simulink model "MotorControl_Bldc"  (R2022a)
settings: Solver=ode4  StartTime=0.0  StopTime=1  FixedStep=Ts/cnt_pTs  RelTol=1e-3
values from neighbouring files (symbols this model uses):
  cnt_pTs = 1000    [motorpara.m]
  Fc = 1/Ts    (= 10000)    [motorpara.m]
  Ki_id = Rs*Fc    (= 4500)    [motorpara.m]
  Ki_iq = Rs*Fc    (= 4500)    [motorpara.m]
  Ki_v = 0.93    [motorpara.m]
  Kp_id = Ls*Fc    (= 4.2)    [motorpara.m]
  Kp_iq = Ls*Fc    (= 4.2)    [motorpara.m]
  Kp_v = 0.05    [motorpara.m]
  Ls = 0.00042    [motorpara.m]
  P = 2    [motorpara.m]
  Rs = 0.45    [motorpara.m]
  SMO_Kslide = 10    [motorpara.m]
  Ts = 1/10000    (= 0.0001)    [motorpara.m]
  V = 12    [motorpara.m]
undefined symbols (not defined in the file or in its folder): DiscIntNeverNeededParam, sigbuilder_block
libraries: nesl_utility x83, fl_lib x67, ee_lib x49, simulink x13, slpidlib x3, mcbplantlib x2, autolibpmsmexterior x1
(part 2 of 4)

== system MotorControl_Bldc/2Phase_D1D1 ==
  alpha : Inport
  m : Inport  Port=2
  N : Inport  Port=3
  Cos : Trigonometry  Operator=cos
  Index Vector : MultiPortSwitch  Inputs=6  DiagnosticForDefault=None  SaturateOnIntegerOverflow=off  InputSameDT=off
  Index Vector1 : MultiPortSwitch  Inputs=6  DiagnosticForDefault=None  SaturateOnIntegerOverflow=off  InputSameDT=off
  Sin : Trigonometry
  c_s : Sum  Inputs=+-
  mcos : Product
  mcos_ : Gain  Gain=-1
  msin : Product
  msin_ : Gain  Gain=-1
  s_c : Gain  Gain=-1
  D1 : Outport
  D2 : Outport  Port=2
  wires:
  Index Vector1/1 -> D2/1
  N/1 -> Index Vector1/1, Index Vector/1
  Index Vector/1 -> D1/1
  alpha/1 -> Sin/1, Cos/1
  Sin/1 -> msin/2
  Cos/1 -> mcos/1
  m/1 -> mcos/2, msin/1
  mcos/1 -> Index Vector/7, Index Vector/3, mcos_/1, c_s/1
  msin/1 -> msin_/1, c_s/2, Index Vector/4, Index Vector1/2
  c_s/1 -> Index Vector1/6, Index Vector/2, s_c/1
  s_c/1 -> Index Vector/5, Index Vector1/3
  mcos_/1 -> Index Vector/6, Index Vector1/4
  msin_/1 -> Index Vector1/7, Index Vector1/5

== system MotorControl_Bldc/2Phase_D1D1_org ==
  alpha : Inport
  m : Inport  Port=2
  N : Inport  Port=3
  Cos : Trigonometry  Operator=cos
  Index Vector : MultiPortSwitch  Inputs=6  DiagnosticForDefault=None  SaturateOnIntegerOverflow=off  InputSameDT=off
  Index Vector1 : MultiPortSwitch  Inputs=6  DiagnosticForDefault=None  SaturateOnIntegerOverflow=off  InputSameDT=off
  Sin : Trigonometry
  c_s : Sum  Inputs=+-
  mcos : Product
  mcos_ : Gain  Gain=-1
  msin : Product
  msin_ : Gain  Gain=-1
  s_c : Gain  Gain=-1
  D1 : Outport
  D2 : Outport  Port=2
  wires:
  Index Vector1/1 -> D2/1
  N/1 -> Index Vector1/1, Index Vector/1
  Index Vector/1 -> D1/1
  alpha/1 -> Sin/1, Cos/1
  Sin/1 -> msin/2
  Cos/1 -> mcos/1
  m/1 -> mcos/2, msin/1
  mcos/1 -> Index Vector/7, Index Vector/3, mcos_/1, c_s/1
  msin/1 -> msin_/1, c_s/2, Index Vector1/7, Index Vector/4, Index Vector1/2
  c_s/1 -> Index Vector1/6, Index Vector/5, Index Vector/2, s_c/1
  s_c/1 -> Index Vector1/3
  mcos_/1 -> Index Vector/6, Index Vector1/4
  msin_/1 -> Index Vector1/5

== system MotorControl_Bldc/2Phase_D1D2 ==
  alpha : Inport
  m : Inport  Port=2
  N : Inport  Port=3
  Cos : Trigonometry  Operator=cos
  Index Vector : MultiPortSwitch  Inputs=6  DiagnosticForDefault=None  SaturateOnIntegerOverflow=off  InputSameDT=off
  Index Vector1 : MultiPortSwitch  Inputs=6  DiagnosticForDefault=None  SaturateOnIntegerOverflow=off  InputSameDT=off
  Sin : Trigonometry
  c_s : Sum  Inputs=+-
  mcos : Product
  mcos_ : Gain  Gain=-1
  msin : Product
  msin_ : Gain  Gain=-1
  s_c : Gain  Gain=-1
  D1 : Outport
  D2 : Outport  Port=2
  wires:
  Index Vector1/1 -> D2/1
  N/1 -> Index Vector1/1, Index Vector/1
  Index Vector/1 -> D1/1
  alpha/1 -> Sin/1, Cos/1
  Sin/1 -> msin/2
  Cos/1 -> mcos/1
  m/1 -> mcos/2, msin/1
  mcos/1 -> Index Vector1/7, Index Vector/3, mcos_/1, c_s/1
  msin/1 -> msin_/1, c_s/2, Index Vector/4, Index Vector1/2
  c_s/1 -> Index Vector1/6, Index Vector/2, s_c/1
  s_c/1 -> Index Vector/5, Index Vector1/3
  mcos_/1 -> Index Vector/6, Index Vector1/4
  msin_/1 -> Index Vector/7, Index Vector1/5

== system MotorControl_Bldc/2Phase_T ==
  note: D1+D2
  note: D1
  note: 1-D1
  note: 1-D1-D2
  N : Inport
  D1 : Inport  Port=2
  D2 : Inport  Port=3
  1_t1 : Sum  Inputs=-+
  1_t2_T2 : Sum  Inputs=-+
  Constant : Constant
  Constant1 : Constant  Value=0
  Index Vector : MultiPortSwitch  Inputs=6  DiagnosticForDefault=None  SaturateOnIntegerOverflow=off  InputSameDT=off
  Index Vector1 : MultiPortSwitch  Inputs=6  DiagnosticForDefault=None  SaturateOnIntegerOverflow=off  InputSameDT=off
  Index Vector2 : MultiPortSwitch  Inputs=6  DiagnosticForDefault=None  SaturateOnIntegerOverflow=off  InputSameDT=off
  T1AT2 : Sum
  Da : Outport
  Db : Outport  Port=2
  Dc : Outport  Port=3
  wires:
  D1/1 -> Index Vector/3, Index Vector2/7, Index Vector1/5, 1_t1/1, T1AT2/1
  D2/1 -> 1_t2_T2/1, T1AT2/2
  N/1 -> Index Vector2/1, Index Vector1/1, Index Vector/1
  Index Vector/1 -> Da/1
  Index Vector1/1 -> Db/1
  Index Vector2/1 -> Dc/1
  Constant/1 -> Index Vector2/6, Index Vector1/4, Index Vector/2, 1_t1/2
  1_t1/1 -> Index Vector1/2, Index Vector/6, Index Vector2/4, 1_t2_T2/2
  T1AT2/1 -> Index Vector/7, Index Vector1/3, Index Vector2/5
  Constant1/1 -> Index Vector1/7, Index Vector/5, Index Vector2/3
  1_t2_T2/1 -> Index Vector2/2, Index Vector1/6, Index Vector/4

== system MotorControl_Bldc/Duty_conver ==
  In1 : Inport
  Constant : Constant  Value=0.5
  Gain : Gain  Gain=1/(5e-5)
  Gain1 : Gain  Gain=-1
  Sum : Sum  Inputs=|+-
  Sum1 : Sum  Inputs=|++
  Out1 : Outport
  wires:
  In1/1 -> Gain/1
  Gain/1 -> Sum/1
  Sum/1 -> Gain1/1
  Gain1/1 -> Sum1/1
  Sum1/1 -> Out1/1
  Constant/1 -> Sum1/2, Sum/2

== system MotorControl_Bldc/Duty_conver1 ==
  In1 : Inport
  Constant : Constant  Value=0.5
  Gain : Gain  Gain=2
  Gain1 : Gain  Gain=-1
  Sum : Sum  Inputs=|+-
  Sum1 : Sum  Inputs=|++
  Out1 : Outport
  wires:
  In1/1 -> Gain/1
  Gain/1 -> Sum/1
  Sum/1 -> Gain1/1
  Gain1/1 -> Sum1/1
  Sum1/1 -> Out1/1
  Constant/1 -> Sum1/2, Sum/2

== system MotorControl_Bldc/Inverse_Park ==
  Vd : Inport
  Vq : Inport  Port=2
  sin_theta : Inport  Port=3
  cos_theta : Inport  Port=4
  Add : Sum  Inputs=+-
  Add1 : Sum
  Product{,1..3} (4 alike) : Product
  Vα : Outport
  Vβ : Outport  Port=2
  wires:
  Vd/1 -> Product3/1, Product/1
  cos_theta/1 -> Product2/2, Product/2
  Vq/1 -> Product2/1, Product1/1
  sin_theta/1 -> Product3/2, Product1/2
  Product/1 -> Add/1
  Product1/1 -> Add/2
  Add/1 -> Vα/1
  Product2/1 -> Add1/1
  Product3/1 -> Add1/2
  Add1/1 -> Vβ/1

== system MotorControl_Bldc/Inverse_Park1 ==
  Vd : Inport
  Vq : Inport  Port=2
  sin_theta : Inport  Port=3
  cos_theta : Inport  Port=4
  Add : Sum  Inputs=+-
  Add1 : Sum
  Product{,1..3} (4 alike) : Product
  Vα : Outport
  Vβ : Outport  Port=2
  wires:
  Vd/1 -> Product3/1, Product/1
  cos_theta/1 -> Product2/2, Product/2
  Vq/1 -> Product2/1, Product1/1
  sin_theta/1 -> Product3/2, Product1/2
  Product/1 -> Add/1
  Product1/1 -> Add/2
  Add/1 -> Vα/1
  Product2/1 -> Add1/1
  Product3/1 -> Add1/2
  Add1/1 -> Vβ/1

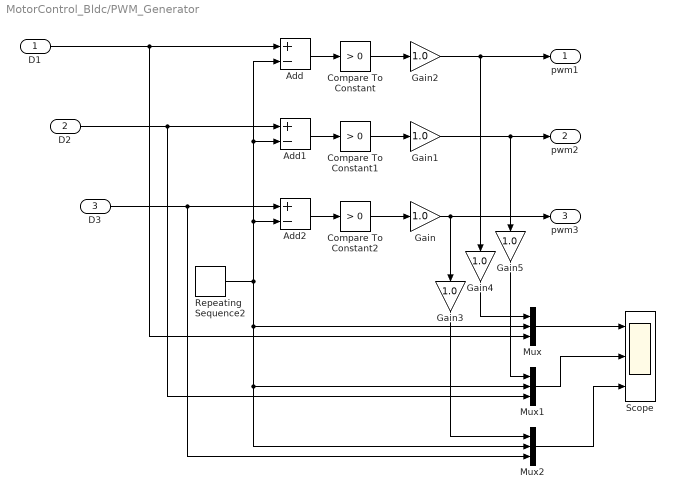
== system MotorControl_Bldc/PWM_Generator ==
  D1 : Inport
  D2 : Inport  Port=2
  D3 : Inport  Port=3
  Add : Sum  Inputs=+-
  Add1 : Sum  Inputs=+-
  Add2 : Sum  Inputs=+-
  Compare To Constant : simulink/Logic and Bit Operations/Compare To Constant  relop=>  const=0  OutDataTypeStr=boolean
  Compare To Constant1 : simulink/Logic and Bit Operations/Compare To Constant  relop=>  const=0  OutDataTypeStr=boolean
  Compare To Constant2 : simulink/Logic and Bit Operations/Compare To Constant  relop=>  const=0  OutDataTypeStr=boolean
  Gain : Gain  Gain=1.0
  Gain1 : Gain  Gain=1.0
  Gain2 : Gain  Gain=1.0
  Gain3 : Gain  Gain=1.0  OutDataTypeStr=double
  Gain4 : Gain  Gain=1.0  OutDataTypeStr=double
  Gain5 : Gain  Gain=1.0  OutDataTypeStr=double
  Mux : Mux  Inputs=3
  Mux1 : Mux  Inputs=3
  Mux2 : Mux  Inputs=3
  Repeating Sequence2 : simulink/Sources/Repeating Sequence  rep_seq_t=[0 Ts/4 Ts/2]  rep_seq_y=[1 0 1]
  Scope : Scope  NumInputPorts=3
  pwm1 : Outport
  pwm2 : Outport  Port=2
  pwm3 : Outport  Port=3
  wires:
  Add2/1 -> Compare To Constant2/1
  Add/1 -> Compare To Constant/1
  Repeating Sequence2/1 -> Mux2/2, Mux1/2, Mux/2, Add2/2, Add1/2, Add/2
  Compare To Constant/1 -> Gain2/1
  Add1/1 -> Compare To Constant1/1
  D2/1 -> Add1/1, Mux1/3
  D3/1 -> Mux2/3, Add2/1
  Compare To Constant2/1 -> Gain/1
  D1/1 -> Mux/3, Add/1
  Compare To Constant1/1 -> Gain1/1
  Gain/1 -> pwm3/1, Gain3/1
  Gain1/1 -> pwm2/1, Gain5/1
  Gain2/1 -> pwm1/1, Gain4/1
  Mux/1 -> Scope/1
  Mux1/1 -> Scope/2
  Mux2/1 -> Scope/3
  Gain3/1 -> Mux2/1
  Gain4/1 -> Mux/1
  Gain5/1 -> Mux1/1

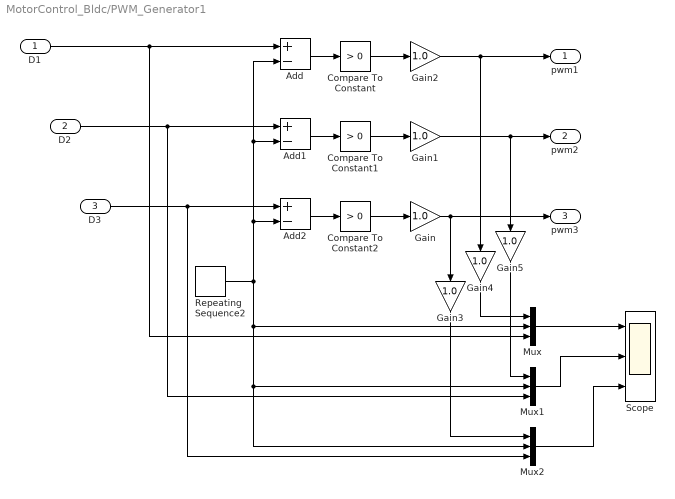
== system MotorControl_Bldc/PWM_Generator1 ==
  D1 : Inport
  D2 : Inport  Port=2
  D3 : Inport  Port=3
  Add : Sum  Inputs=+-
  Add1 : Sum  Inputs=+-
  Add2 : Sum  Inputs=+-
  Compare To Constant : simulink/Logic and Bit Operations/Compare To Constant  relop=>  const=0  OutDataTypeStr=boolean
  Compare To Constant1 : simulink/Logic and Bit Operations/Compare To Constant  relop=>  const=0  OutDataTypeStr=boolean
  Compare To Constant2 : simulink/Logic and Bit Operations/Compare To Constant  relop=>  const=0  OutDataTypeStr=boolean
  Gain : Gain  Gain=1.0
  Gain1 : Gain  Gain=1.0
  Gain2 : Gain  Gain=1.0
  Gain3 : Gain  Gain=1.0  OutDataTypeStr=double
  Gain4 : Gain  Gain=1.0  OutDataTypeStr=double
  Gain5 : Gain  Gain=1.0  OutDataTypeStr=double
  Mux : Mux  Inputs=3
  Mux1 : Mux  Inputs=3
  Mux2 : Mux  Inputs=3
  Repeating Sequence2 : simulink/Sources/Repeating Sequence  rep_seq_t=[0 Ts/4 Ts/2]  rep_seq_y=[1 0 1]
  Scope : Scope  NumInputPorts=3
  pwm1 : Outport
  pwm2 : Outport  Port=2
  pwm3 : Outport  Port=3
  wires:
  Add2/1 -> Compare To Constant2/1
  Add/1 -> Compare To Constant/1
  Repeating Sequence2/1 -> Mux2/2, Mux1/2, Mux/2, Add2/2, Add1/2, Add/2
  Compare To Constant/1 -> Gain2/1
  Add1/1 -> Compare To Constant1/1
  D2/1 -> Add1/1, Mux1/3
  D3/1 -> Mux2/3, Add2/1
  Compare To Constant2/1 -> Gain/1
  D1/1 -> Mux/3, Add/1
  Compare To Constant1/1 -> Gain1/1
  Gain/1 -> pwm3/1, Gain3/1
  Gain1/1 -> pwm2/1, Gain5/1
  Gain2/1 -> pwm1/1, Gain4/1
  Mux/1 -> Scope/1
  Mux1/1 -> Scope/2
  Mux2/1 -> Scope/3
  Gain3/1 -> Mux2/1
  Gain4/1 -> Mux/1
  Gain5/1 -> Mux1/1

== system MotorControl_Bldc/Park ==
  Iα : Inport
  Iβ : Inport  Port=2
  Sin_Theta : Inport  Port=3
  Cos_Theta : Inport  Port=4
  Add : Sum
  Add1 : Sum  Inputs=-+
  Product{,1..3} (4 alike) : Product
  Id : Outport
  Iq : Outport  Port=2
  wires:
  Cos_Theta/1 -> Product3/1, Product/2
  Add/1 -> Id/1
  Iβ/1 -> Product1/1, Product3/2
  Sin_Theta/1 -> Product2/1, Product1/2
  Product/1 -> Add/1
  Product1/1 -> Add/2
  Iα/1 -> Product/1, Product2/2
  Product2/1 -> Add1/1
  Product3/1 -> Add1/2
  Add1/1 -> Iq/1

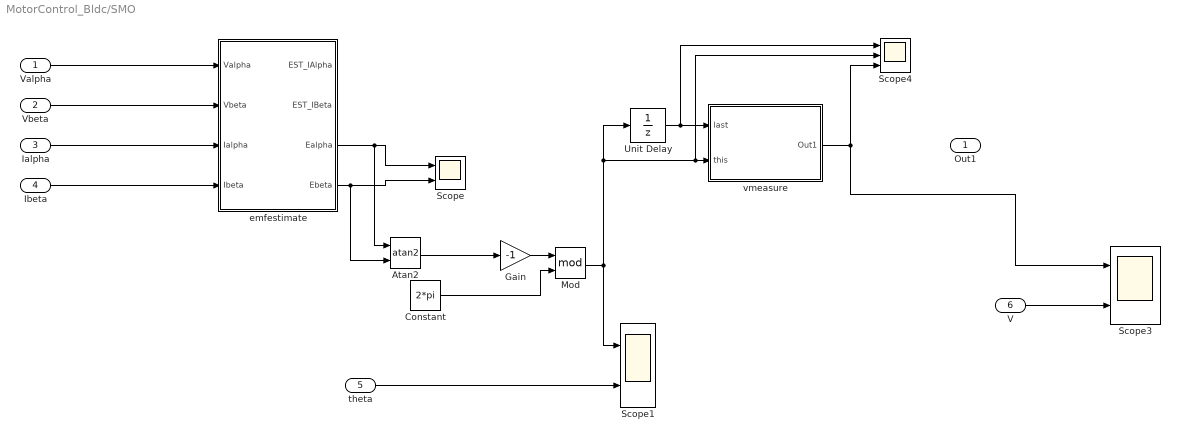
== system MotorControl_Bldc/SMO ==
  Valpha : Inport
  Vbeta : Inport  Port=2
  Ialpha : Inport  Port=3
  Ibeta : Inport  Port=4
  theta : Inport  Port=5
  V : Inport  Port=6
  Atan2 : Trigonometry  Operator=atan2
  Constant : Constant  Value=2*pi
  Gain : Gain  Gain=-1
  Mod : Math  Operator=mod
  Scope : Scope  NumInputPorts=2
  Scope1 : Scope  NumInputPorts=2
  Scope3 : Scope  NumInputPorts=2
  Scope4 : Scope  NumInputPorts=3
  Unit Delay : UnitDelay  SampleTime=Ts  HasFrameUpgradeWarning=on
  emfestimate : Subsystem
  vmeasure : Subsystem
  Out1 : Outport
  wires:
  Valpha/1 -> emfestimate/1(Valpha)
  Vbeta/1 -> emfestimate/2(Vbeta)
  Ialpha/1 -> emfestimate/3(Ialpha)
  Ibeta/1 -> emfestimate/4(Ibeta)
  emfestimate/3(Ealpha) -> Atan2/1, Scope/1
  emfestimate/4(Ebeta) -> Atan2/2, Scope/2
  theta/1 -> Scope1/2
  Atan2/1 -> Gain/1
  Gain/1 -> Mod/1
  Constant/1 -> Mod/2
  Mod/1 -> Scope4/2, vmeasure/2(this), Unit Delay/1, Scope1/1
  Unit Delay/1 -> Scope4/1, vmeasure/1(last)
  vmeasure/1(Out1) -> Scope4/3, Scope3/1
  V/1 -> Scope3/2

== system MotorControl_Bldc/SVPWM ==
  Vα : Inport
  Vβ : Inport  Port=2
  Vbus : Inport  Port=3
  TS : Inport  Port=4
  Constant : Constant  Value=Ts
  Sector : Subsystem
  Subsystem : Subsystem
  T1T2 : Subsystem
  XYZ : Subsystem
  Ta : Outport
  Tb : Outport  Port=2
  Tc : Outport  Port=3
  Sector_O : Outport  Port=4
  wires:
  Vα/1 -> XYZ/1(Vα), Sector/1(Vα)
  Sector/1(N) -> Sector_O/1, T1T2/1(N), Subsystem/1(N)
  TS/1 -> XYZ/4(TS)
  Vbus/1 -> XYZ/3(Vbus)
  Vβ/1 -> Sector/2(Vβ), XYZ/2(Vβ)
  XYZ/1(X) -> T1T2/2(X)
  XYZ/2(Y) -> T1T2/3(Y)
  XYZ/3(Z) -> T1T2/4(Z)
  T1T2/1(T1) -> Subsystem/2(T1)
  T1T2/2(T2) -> Subsystem/3(T2)
  Constant/1 -> Subsystem/4(TS)
  Subsystem/1(Ta) -> Ta/1
  Subsystem/2(Tb) -> Tb/1
  Subsystem/3(Tc) -> Tc/1

== system MotorControl_Bldc/SVPWM1 ==
  Vα : Inport
  Vβ : Inport  Port=2
  Vbus : Inport  Port=3
  TS : Inport  Port=4
  Constant : Constant
  Sector : Subsystem
  Subsystem : Subsystem
  T1T2 : Subsystem
  XYZ : Subsystem
  Ta : Outport
  Tb : Outport  Port=2
  Tc : Outport  Port=3
  wires:
  Vα/1 -> XYZ/1(Vα), Sector/1(Vα)
  Sector/1(N) -> T1T2/1(N), Subsystem/1(N)
  TS/1 -> XYZ/4(TS)
  Vbus/1 -> XYZ/3(Vbus)
  Vβ/1 -> Sector/2(Vβ), XYZ/2(Vβ)
  XYZ/1(X) -> T1T2/2(X)
  XYZ/2(Y) -> T1T2/3(Y)
  XYZ/3(Z) -> T1T2/4(Z)
  T1T2/1(T1) -> Subsystem/2(T1)
  T1T2/2(T2) -> Subsystem/3(T2)
  Constant/1 -> Subsystem/4(TS)
  Subsystem/1(Ta) -> Ta/1
  Subsystem/2(Tb) -> Tb/1
  Subsystem/3(Tc) -> Tc/1

== system MotorControl_Bldc/Sector1 ==
  note: ALPHA 应该在0到2Pi之间
  Alpha : Inport
  Add2 : Sum  Inputs=++++++
  Constant : Constant
  Constant1 : Constant  Value=0
  Switch1 : Switch  Criteria=u2 > Threshold  Threshold=pi/4  SaturateOnIntegerOverflow=off  InputSameDT=off
  Switch2 : Switch  Criteria=u2 > Threshold  Threshold=pi/2  SaturateOnIntegerOverflow=off  InputSameDT=off
  Switch3 : Switch  Criteria=u2 > Threshold  Threshold=pi  SaturateOnIntegerOverflow=off  InputSameDT=off
  Switch4 : Switch  Criteria=u2 > Threshold  Threshold=5*pi/4  SaturateOnIntegerOverflow=off  InputSameDT=off
  Switch5 : Switch  Criteria=u2 > Threshold  Threshold=3*pi/2  SaturateOnIntegerOverflow=off  InputSameDT=off
  pid4 : Switch  SaturateOnIntegerOverflow=off  InputSameDT=off
  N : Outport
  wires:
  pid4/1 -> Add2/1
  Switch1/1 -> Add2/2
  Switch2/1 -> Add2/3
  Add2/1 -> N/1
  Constant/1 -> Switch5/1, Switch4/1, Switch3/1, Switch2/1, Switch1/1, pid4/1
  Switch3/1 -> Add2/4
  Switch4/1 -> Add2/5
  Switch5/1 -> Add2/6
  Constant1/1 -> Switch4/3, Switch3/3, Switch2/3, Switch1/3, pid4/3, Switch5/3
  Alpha/1 -> Switch4/2, Switch5/2, Switch3/2, Switch2/2, Switch1/2, pid4/2

== system MotorControl_Bldc/Sector2 ==
  Vα : Inport
  Vβ : Inport  Port=2
  Add : Sum  Inputs=+-
  Add1 : Sum  Inputs=--
  Add2 : Sum  Inputs=+++
  Constant : Constant
  Constant1 : Constant  Value=0
  Gain : Gain  Gain=sqrt(3)
  Gain1 : Gain  Gain=4
  Gain2 : Gain  Gain=2
  Gain3 : Gain
  Switch : Switch  Criteria=u2 > Threshold  SaturateOnIntegerOverflow=off  InputSameDT=off
  Switch1 : Switch  Criteria=u2 > Threshold  SaturateOnIntegerOverflow=off  InputSameDT=off
  Switch2 : Switch  Criteria=u2 > Threshold  SaturateOnIntegerOverflow=off  InputSameDT=off
  N : Outport
  wires:
  Vα/1 -> Gain/1
  Gain/1 -> Add1/1, Add/1
  Vβ/1 -> Add1/2, Switch/2, Add/2
  Add/1 -> Switch1/2
  Add1/1 -> Switch2/2
  Constant1/1 -> Switch/3, Switch1/3, Switch2/3
  Constant/1 -> Switch2/1, Switch1/1, Switch/1
  Switch/1 -> Gain3/1
  Switch1/1 -> Gain2/1
  Switch2/1 -> Gain1/1
  Gain3/1 -> Add2/1
  Gain2/1 -> Add2/2
  Gain1/1 -> Add2/3
  Add2/1 -> N/1

== system MotorControl_Bldc/Sensing trq1 ==
  MRRef : fl_lib/Mechanical/Rotational Elements/Mechanical Rotational Reference
      settings: SourceProductBaseCode=PW,SS,VE
  Motion Sensor : fl_lib/Mechanical/Mechanical Sensors/Ideal Rotational Motion Sensor  wrap_angle=simscape.enum.onoff.off  offset=0 deg
      settings: SourceProductBaseCode=PW,SS,VE
  PS-Simulink Converter1 : nesl_utility/PS-Simulink Converter  PhysicalDomain=network_engine_domain  SubClassName=ps_output  LeftPortType=input  RightPortType=output  PseudoPeriodic=off  Frequencies=[]  VectorFormat=1-D array  Unit=rad/s  AffineConversion=off
      settings: SourceProductBaseCode=SS,PW,VE
  PS-Simulink Converter3 : nesl_utility/PS-Simulink Converter  PhysicalDomain=network_engine_domain  SubClassName=ps_output  LeftPortType=input  RightPortType=output  PseudoPeriodic=off  Frequencies=[]  VectorFormat=1-D array  Unit=N*m  AffineConversion=off
      settings: SourceProductBaseCode=SS,PW,VE
  Torque Sensor : fl_lib/Mechanical/Mechanical Sensors/Ideal Torque Sensor
      settings: SourceProductBaseCode=PW,SS,VE
  R : PMIOPort  Side=Left
  C : PMIOPort  Port=2  Side=Right
  Tq : Outport
  w : Outport  Port=2
  wires:
  PS-Simulink Converter3/1 -> Tq/1
  PS-Simulink Converter1/1 -> w/1
  connections:
  Torque Sensor/RConn1 -- Motion Sensor/LConn1 -- C/RConn1
  Torque Sensor/RConn2 -- PS-Simulink Converter3/LConn1
  Torque Sensor/LConn1 -- R/RConn1
  MRRef/LConn1 -- Motion Sensor/RConn1
  Motion Sensor/RConn2 -- PS-Simulink Converter1/LConn1

== system MotorControl_Bldc/Sensing trq3 ==
  MRRef : fl_lib/Mechanical/Rotational Elements/Mechanical Rotational Reference
      settings: SourceProductBaseCode=PW,SS,VE
  Motion Sensor : fl_lib/Mechanical/Mechanical Sensors/Ideal Rotational Motion Sensor  wrap_angle=simscape.enum.onoff.off  offset=0 deg
      settings: SourceProductBaseCode=PW,SS,VE
  PS-Simulink Converter1 : nesl_utility/PS-Simulink Converter  PhysicalDomain=network_engine_domain  SubClassName=ps_output  LeftPortType=input  RightPortType=output  PseudoPeriodic=off  Frequencies=[]  VectorFormat=1-D array  Unit=rad/s  AffineConversion=off
      settings: SourceProductBaseCode=SS,PW,VE
  PS-Simulink Converter3 : nesl_utility/PS-Simulink Converter  PhysicalDomain=network_engine_domain  SubClassName=ps_output  LeftPortType=input  RightPortType=output  PseudoPeriodic=off  Frequencies=[]  VectorFormat=1-D array  Unit=N*m  AffineConversion=off
      settings: SourceProductBaseCode=SS,PW,VE
  Torque Sensor : fl_lib/Mechanical/Mechanical Sensors/Ideal Torque Sensor
      settings: SourceProductBaseCode=PW,SS,VE
  R : PMIOPort  Side=Left
  C : PMIOPort  Port=2  Side=Right
  Tq : Outport
  w : Outport  Port=2
  wires:
  PS-Simulink Converter3/1 -> Tq/1
  PS-Simulink Converter1/1 -> w/1
  connections:
  Torque Sensor/RConn1 -- Motion Sensor/LConn1 -- C/RConn1
  Torque Sensor/RConn2 -- PS-Simulink Converter3/LConn1
  Torque Sensor/LConn1 -- R/RConn1
  MRRef/LConn1 -- Motion Sensor/RConn1
  Motion Sensor/RConn2 -- PS-Simulink Converter1/LConn1

== system MotorControl_Bldc/Signal Builder ==
  Demux : Demux  Tag=STV Demux  Outputs=1
      settings: DisplayOption=none
  FromWs : FromWorkspace  Tag=STV FromWs  VariableName=tuvar
      SigBuilderData=|
      | common.afterFinalStr = 'Extrapolate'
      | common.sampleTime = 0
      | dataSet.timeRange = [0 10]
      | dataSet.name = 'Group 1'
      | sbobj.Groups.Name = 'Group 1'
      | sbobj.Groups.Signals.Name = 'Signal 1'
      | sbobj.Groups.Signals.XData = [0 0.3 0.4 0.6 0.9 10]
      | sbobj.Groups.Signals.YData = [0.29 0.315 0.59 0.59 0.3 0.045]
  Signal 1 : Outport  Tag=STV Outport
  wires:
  Demux/1 -> Signal 1/1
  FromWs/1 -> Demux/1

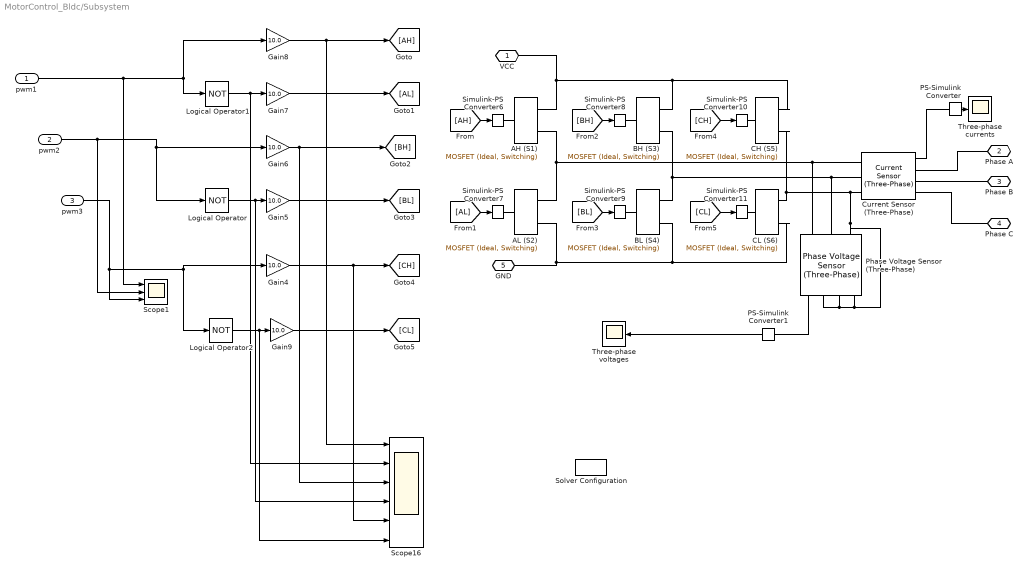
== system MotorControl_Bldc/Subsystem ==
  pwm1 : Inport
  pwm2 : Inport  Port=2
  pwm3 : Inport  Port=3
  AH (S1) : ee_lib/Semiconductors & Converters/MOSFET (Ideal, Switching)  Rds=0.01 Ohm  Goff=1e-6 1/Ohm  Vth=0.5 V  diode_param=2  diode_Vf=0.1 V  diode_Ron=0.001 Ohm  diode_Goff=1e-5 1/Ohm  diode_C=50e-9 F  diode_iRM=-235 A  diode_iF=300 A  diode_idot=-50 A/us  diode_trr_param=1  diode_trr_factor=3  diode_trr=15 us  diode_Qrr=1500 s*uA  thermal_loss_option=ee.enum.converters.thermalLossOption.constantvalues  Von_data=[0, 1.1, 1.3, 1.45, 1.75, 2.25, 2.7; 0, 1, 1.15, 1.35, 1.7, 2.35, 3] V  Tj=[298.15, 398.15] K  Iout_data=[0, 10, 50, 100, 200, 400, 600] A  Eon_data=[0, .29, 1.43, 2.86, 5.71, 13.14, 22.86; 0, .57, 2.63, 5.14, 10.29, 20.57, 30.29] * 1e-3 J  Eoff_data=[0, .21, 1.07, 2.14, 4.29, 9.86, 17.14; 0, .43, 1.97, 3.86, 7.71, 15.43, 22.71] * 1e-3 J  Tj_loss=[298.15, 398.15] K  Iout_data_loss=[0, 10, 50, 100, 200, 400, 600] A  Eon_scalar=22.86e-3 J  Eoff_scalar=17.14e-3 J  Voff=300 V  Iout_scalar=600 A  diodeModelType=ee.enum.converters.diodeModelType.pwl  diodeTableType=ee.enum.diode.tableType.IfMat  diode_IfMat=[.07, .12, .19, 1.75, 4.24, 7.32, 11.2; .16, .3, .72, 2.14, 4.02, 6.35, 9.12] A  diode_VfMat=[.9, 1.15, 1.25, 1.5, 1.75, 2.17, 2.6, 2.85; .58, .68, .75, 1.1, 1.38, 1.77, 2.27, 2.7] V  diode_TjVec=[25, 125] degC  diode_VfVec=[.5, .7, .9, 1.3, 1.7, 2.1, 2.5] V  diode_IfVec=[.1, .2, .5, 1, 2, 4, 7, 10] A  diode_Vr=-600 V  diode_Ls=150 nH  diode_Erec=0.03 J  thermal_network_parameterization=ee.enum.thermalNetworkTopology.external  Rth=[.03, .2] K/W  Rth_Cauer=[.03, .1, .2] K/W  Rth_Foster=[.03, .2] K/W  thermal_mass_parameterization=ee.enum.thermalNetwork.timeconstant  thermal_mass=[3, 25] J/K  thermal_mass_Cauer=[3, 10, 25] J/K  thermal_mass_Foster=[33, 50] J/K  thermal_time_constant=[.1, 5] s  thermal_time_constant_Cauer=[.1, 1, 5] s  thermal_time_constant_Foster=[1, 10] s  thermal_mass_initial_temperatures=[25, 25] degC  thermal_mass_initial_temperatures_Cauer=[25, 25, 25] degC  junction_thermal_mass=0.1 J/K  steadyState_Foster=simscape.enum.onoff.on  Tvec_initial_Foster=[25, 25, 25, 25] degC  no_thermal_network=0  junction_temperature_specify=off  junction_temperature_priority=None  junction_temperature=25 degC  junction_temperature_nominal_specify=off  junction_temperature_nominal_unit=degC  junction_temperature_nominal_value=1  vT_specify=off  vT_priority=None  vT=0 V  vT_nominal_specify=off  vT_nominal_unit=V  vT_nominal_value=1  Qj_specify=off  Qj_priority=None  Qj=0 W  Qj_nominal_specify=off  Qj_nominal_unit=W  Qj_nominal_value=1
  AL (S2) : ee_lib/Semiconductors & Converters/MOSFET (Ideal, Switching)  Rds=0.01 Ohm  Goff=1e-6 1/Ohm  Vth=0.5 V  diode_param=2  diode_Vf=0.1 V  diode_Ron=0.001 Ohm  diode_Goff=1e-5 1/Ohm  diode_C=50e-9 F  diode_iRM=-235 A  diode_iF=300 A  diode_idot=-50 A/us  diode_trr_param=1  diode_trr_factor=3  diode_trr=15 us  diode_Qrr=1500 s*uA  thermal_loss_option=ee.enum.converters.thermalLossOption.constantvalues  Von_data=[0, 1.1, 1.3, 1.45, 1.75, 2.25, 2.7; 0, 1, 1.15, 1.35, 1.7, 2.35, 3] V  Tj=[298.15, 398.15] K  Iout_data=[0, 10, 50, 100, 200, 400, 600] A  Eon_data=[0, .29, 1.43, 2.86, 5.71, 13.14, 22.86; 0, .57, 2.63, 5.14, 10.29, 20.57, 30.29] * 1e-3 J  Eoff_data=[0, .21, 1.07, 2.14, 4.29, 9.86, 17.14; 0, .43, 1.97, 3.86, 7.71, 15.43, 22.71] * 1e-3 J  Tj_loss=[298.15, 398.15] K  Iout_data_loss=[0, 10, 50, 100, 200, 400, 600] A  Eon_scalar=22.86e-3 J  Eoff_scalar=17.14e-3 J  Voff=300 V  Iout_scalar=600 A  diodeModelType=ee.enum.converters.diodeModelType.pwl  diodeTableType=ee.enum.diode.tableType.IfMat  diode_IfMat=[.07, .12, .19, 1.75, 4.24, 7.32, 11.2; .16, .3, .72, 2.14, 4.02, 6.35, 9.12] A  diode_VfMat=[.9, 1.15, 1.25, 1.5, 1.75, 2.17, 2.6, 2.85; .58, .68, .75, 1.1, 1.38, 1.77, 2.27, 2.7] V  diode_TjVec=[25, 125] degC  diode_VfVec=[.5, .7, .9, 1.3, 1.7, 2.1, 2.5] V  diode_IfVec=[.1, .2, .5, 1, 2, 4, 7, 10] A  diode_Vr=-600 V  diode_Ls=150 nH  diode_Erec=0.03 J  thermal_network_parameterization=ee.enum.thermalNetworkTopology.external  Rth=[.03, .2] K/W  Rth_Cauer=[.03, .1, .2] K/W  Rth_Foster=[.03, .2] K/W  thermal_mass_parameterization=ee.enum.thermalNetwork.timeconstant  thermal_mass=[3, 25] J/K  thermal_mass_Cauer=[3, 10, 25] J/K  thermal_mass_Foster=[33, 50] J/K  thermal_time_constant=[.1, 5] s  thermal_time_constant_Cauer=[.1, 1, 5] s  thermal_time_constant_Foster=[1, 10] s  thermal_mass_initial_temperatures=[25, 25] degC  thermal_mass_initial_temperatures_Cauer=[25, 25, 25] degC  junction_thermal_mass=0.1 J/K  steadyState_Foster=simscape.enum.onoff.on  Tvec_initial_Foster=[25, 25, 25, 25] degC  no_thermal_network=0  junction_temperature_specify=off  junction_temperature_priority=None  junction_temperature=25 degC  junction_temperature_nominal_specify=off  junction_temperature_nominal_unit=degC  junction_temperature_nominal_value=1  vT_specify=off  vT_priority=None  vT=0 V  vT_nominal_specify=off  vT_nominal_unit=V  vT_nominal_value=1  Qj_specify=off  Qj_priority=None  Qj=0 W  Qj_nominal_specify=off  Qj_nominal_unit=W  Qj_nominal_value=1
  BH (S3) : ee_lib/Semiconductors & Converters/MOSFET (Ideal, Switching)  Rds=0.01 Ohm  Goff=1e-6 1/Ohm  Vth=0.5 V  diode_param=2  diode_Vf=0.1 V  diode_Ron=0.001 Ohm  diode_Goff=1e-5 1/Ohm  diode_C=50e-9 F  diode_iRM=-235 A  diode_iF=300 A  diode_idot=-50 A/us  diode_trr_param=1  diode_trr_factor=3  diode_trr=15 us  diode_Qrr=1500 s*uA  thermal_loss_option=ee.enum.converters.thermalLossOption.constantvalues  Von_data=[0, 1.1, 1.3, 1.45, 1.75, 2.25, 2.7; 0, 1, 1.15, 1.35, 1.7, 2.35, 3] V  Tj=[298.15, 398.15] K  Iout_data=[0, 10, 50, 100, 200, 400, 600] A  Eon_data=[0, .29, 1.43, 2.86, 5.71, 13.14, 22.86; 0, .57, 2.63, 5.14, 10.29, 20.57, 30.29] * 1e-3 J  Eoff_data=[0, .21, 1.07, 2.14, 4.29, 9.86, 17.14; 0, .43, 1.97, 3.86, 7.71, 15.43, 22.71] * 1e-3 J  Tj_loss=[298.15, 398.15] K  Iout_data_loss=[0, 10, 50, 100, 200, 400, 600] A  Eon_scalar=22.86e-3 J  Eoff_scalar=17.14e-3 J  Voff=300 V  Iout_scalar=600 A  diodeModelType=ee.enum.converters.diodeModelType.pwl  diodeTableType=ee.enum.diode.tableType.IfMat  diode_IfMat=[.07, .12, .19, 1.75, 4.24, 7.32, 11.2; .16, .3, .72, 2.14, 4.02, 6.35, 9.12] A  diode_VfMat=[.9, 1.15, 1.25, 1.5, 1.75, 2.17, 2.6, 2.85; .58, .68, .75, 1.1, 1.38, 1.77, 2.27, 2.7] V  diode_TjVec=[25, 125] degC  diode_VfVec=[.5, .7, .9, 1.3, 1.7, 2.1, 2.5] V  diode_IfVec=[.1, .2, .5, 1, 2, 4, 7, 10] A  diode_Vr=-600 V  diode_Ls=150 nH  diode_Erec=0.03 J  thermal_network_parameterization=ee.enum.thermalNetworkTopology.external  Rth=[.03, .2] K/W  Rth_Cauer=[.03, .1, .2] K/W  Rth_Foster=[.03, .2] K/W  thermal_mass_parameterization=ee.enum.thermalNetwork.timeconstant  thermal_mass=[3, 25] J/K  thermal_mass_Cauer=[3, 10, 25] J/K  thermal_mass_Foster=[33, 50] J/K  thermal_time_constant=[.1, 5] s  thermal_time_constant_Cauer=[.1, 1, 5] s  thermal_time_constant_Foster=[1, 10] s  thermal_mass_initial_temperatures=[25, 25] degC  thermal_mass_initial_temperatures_Cauer=[25, 25, 25] degC  junction_thermal_mass=0.1 J/K  steadyState_Foster=simscape.enum.onoff.on  Tvec_initial_Foster=[25, 25, 25, 25] degC  no_thermal_network=0  junction_temperature_specify=off  junction_temperature_priority=None  junction_temperature=25 degC  junction_temperature_nominal_specify=off  junction_temperature_nominal_unit=degC  junction_temperature_nominal_value=1  vT_specify=off  vT_priority=None  vT=0 V  vT_nominal_specify=off  vT_nominal_unit=V  vT_nominal_value=1  Qj_specify=off  Qj_priority=None  Qj=0 W  Qj_nominal_specify=off  Qj_nominal_unit=W  Qj_nominal_value=1
  BL (S4) : ee_lib/Semiconductors & Converters/MOSFET (Ideal, Switching)  Rds=0.01 Ohm  Goff=1e-6 1/Ohm  Vth=0.5 V  diode_param=2  diode_Vf=0.1 V  diode_Ron=0.001 Ohm  diode_Goff=1e-5 1/Ohm  diode_C=50e-9 F  diode_iRM=-235 A  diode_iF=300 A  diode_idot=-50 A/us  diode_trr_param=1  diode_trr_factor=3  diode_trr=15 us  diode_Qrr=1500 s*uA  thermal_loss_option=ee.enum.converters.thermalLossOption.constantvalues  Von_data=[0, 1.1, 1.3, 1.45, 1.75, 2.25, 2.7; 0, 1, 1.15, 1.35, 1.7, 2.35, 3] V  Tj=[298.15, 398.15] K  Iout_data=[0, 10, 50, 100, 200, 400, 600] A  Eon_data=[0, .29, 1.43, 2.86, 5.71, 13.14, 22.86; 0, .57, 2.63, 5.14, 10.29, 20.57, 30.29] * 1e-3 J  Eoff_data=[0, .21, 1.07, 2.14, 4.29, 9.86, 17.14; 0, .43, 1.97, 3.86, 7.71, 15.43, 22.71] * 1e-3 J  Tj_loss=[298.15, 398.15] K  Iout_data_loss=[0, 10, 50, 100, 200, 400, 600] A  Eon_scalar=22.86e-3 J  Eoff_scalar=17.14e-3 J  Voff=300 V  Iout_scalar=600 A  diodeModelType=ee.enum.converters.diodeModelType.pwl  diodeTableType=ee.enum.diode.tableType.IfMat  diode_IfMat=[.07, .12, .19, 1.75, 4.24, 7.32, 11.2; .16, .3, .72, 2.14, 4.02, 6.35, 9.12] A  diode_VfMat=[.9, 1.15, 1.25, 1.5, 1.75, 2.17, 2.6, 2.85; .58, .68, .75, 1.1, 1.38, 1.77, 2.27, 2.7] V  diode_TjVec=[25, 125] degC  diode_VfVec=[.5, .7, .9, 1.3, 1.7, 2.1, 2.5] V  diode_IfVec=[.1, .2, .5, 1, 2, 4, 7, 10] A  diode_Vr=-600 V  diode_Ls=150 nH  diode_Erec=0.03 J  thermal_network_parameterization=ee.enum.thermalNetworkTopology.external  Rth=[.03, .2] K/W  Rth_Cauer=[.03, .1, .2] K/W  Rth_Foster=[.03, .2] K/W  thermal_mass_parameterization=ee.enum.thermalNetwork.timeconstant  thermal_mass=[3, 25] J/K  thermal_mass_Cauer=[3, 10, 25] J/K  thermal_mass_Foster=[33, 50] J/K  thermal_time_constant=[.1, 5] s  thermal_time_constant_Cauer=[.1, 1, 5] s  thermal_time_constant_Foster=[1, 10] s  thermal_mass_initial_temperatures=[25, 25] degC  thermal_mass_initial_temperatures_Cauer=[25, 25, 25] degC  junction_thermal_mass=0.1 J/K  steadyState_Foster=simscape.enum.onoff.on  Tvec_initial_Foster=[25, 25, 25, 25] degC  no_thermal_network=0  junction_temperature_specify=off  junction_temperature_priority=None  junction_temperature=25 degC  junction_temperature_nominal_specify=off  junction_temperature_nominal_unit=degC  junction_temperature_nominal_value=1  vT_specify=off  vT_priority=None  vT=0 V  vT_nominal_specify=off  vT_nominal_unit=V  vT_nominal_value=1  Qj_specify=off  Qj_priority=None  Qj=0 W  Qj_nominal_specify=off  Qj_nominal_unit=W  Qj_nominal_value=1
  CH (S5) : ee_lib/Semiconductors & Converters/MOSFET (Ideal, Switching)  Rds=0.01 Ohm  Goff=1e-6 1/Ohm  Vth=0.5 V  diode_param=2  diode_Vf=0.1 V  diode_Ron=0.001 Ohm  diode_Goff=1e-5 1/Ohm  diode_C=50e-9 F  diode_iRM=-235 A  diode_iF=300 A  diode_idot=-50 A/us  diode_trr_param=1  diode_trr_factor=3  diode_trr=15 us  diode_Qrr=1500 s*uA  thermal_loss_option=ee.enum.converters.thermalLossOption.constantvalues  Von_data=[0, 1.1, 1.3, 1.45, 1.75, 2.25, 2.7; 0, 1, 1.15, 1.35, 1.7, 2.35, 3] V  Tj=[298.15, 398.15] K  Iout_data=[0, 10, 50, 100, 200, 400, 600] A  Eon_data=[0, .29, 1.43, 2.86, 5.71, 13.14, 22.86; 0, .57, 2.63, 5.14, 10.29, 20.57, 30.29] * 1e-3 J  Eoff_data=[0, .21, 1.07, 2.14, 4.29, 9.86, 17.14; 0, .43, 1.97, 3.86, 7.71, 15.43, 22.71] * 1e-3 J  Tj_loss=[298.15, 398.15] K  Iout_data_loss=[0, 10, 50, 100, 200, 400, 600] A  Eon_scalar=22.86e-3 J  Eoff_scalar=17.14e-3 J  Voff=300 V  Iout_scalar=600 A  diodeModelType=ee.enum.converters.diodeModelType.pwl  diodeTableType=ee.enum.diode.tableType.IfMat  diode_IfMat=[.07, .12, .19, 1.75, 4.24, 7.32, 11.2; .16, .3, .72, 2.14, 4.02, 6.35, 9.12] A  diode_VfMat=[.9, 1.15, 1.25, 1.5, 1.75, 2.17, 2.6, 2.85; .58, .68, .75, 1.1, 1.38, 1.77, 2.27, 2.7] V  diode_TjVec=[25, 125] degC  diode_VfVec=[.5, .7, .9, 1.3, 1.7, 2.1, 2.5] V  diode_IfVec=[.1, .2, .5, 1, 2, 4, 7, 10] A  diode_Vr=-600 V  diode_Ls=150 nH  diode_Erec=0.03 J  thermal_network_parameterization=ee.enum.thermalNetworkTopology.external  Rth=[.03, .2] K/W  Rth_Cauer=[.03, .1, .2] K/W  Rth_Foster=[.03, .2] K/W  thermal_mass_parameterization=ee.enum.thermalNetwork.timeconstant  thermal_mass=[3, 25] J/K  thermal_mass_Cauer=[3, 10, 25] J/K  thermal_mass_Foster=[33, 50] J/K  thermal_time_constant=[.1, 5] s  thermal_time_constant_Cauer=[.1, 1, 5] s  thermal_time_constant_Foster=[1, 10] s  thermal_mass_initial_temperatures=[25, 25] degC  thermal_mass_initial_temperatures_Cauer=[25, 25, 25] degC  junction_thermal_mass=0.1 J/K  steadyState_Foster=simscape.enum.onoff.on  Tvec_initial_Foster=[25, 25, 25, 25] degC  no_thermal_network=0  junction_temperature_specify=off  junction_temperature_priority=None  junction_temperature=25 degC  junction_temperature_nominal_specify=off  junction_temperature_nominal_unit=degC  junction_temperature_nominal_value=1  vT_specify=off  vT_priority=None  vT=0 V  vT_nominal_specify=off  vT_nominal_unit=V  vT_nominal_value=1  Qj_specify=off  Qj_priority=None  Qj=0 W  Qj_nominal_specify=off  Qj_nominal_unit=W  Qj_nominal_value=1
  CL (S6) : ee_lib/Semiconductors & Converters/MOSFET (Ideal, Switching)  Rds=0.01 Ohm  Goff=1e-6 1/Ohm  Vth=0.5 V  diode_param=2  diode_Vf=0.1 V  diode_Ron=0.001 Ohm  diode_Goff=1e-5 1/Ohm  diode_C=50e-9 F  diode_iRM=-235 A  diode_iF=300 A  diode_idot=-50 A/us  diode_trr_param=1  diode_trr_factor=3  diode_trr=15 us  diode_Qrr=1500 s*uA  thermal_loss_option=ee.enum.converters.thermalLossOption.constantvalues  Von_data=[0, 1.1, 1.3, 1.45, 1.75, 2.25, 2.7; 0, 1, 1.15, 1.35, 1.7, 2.35, 3] V  Tj=[298.15, 398.15] K  Iout_data=[0, 10, 50, 100, 200, 400, 600] A  Eon_data=[0, .29, 1.43, 2.86, 5.71, 13.14, 22.86; 0, .57, 2.63, 5.14, 10.29, 20.57, 30.29] * 1e-3 J  Eoff_data=[0, .21, 1.07, 2.14, 4.29, 9.86, 17.14; 0, .43, 1.97, 3.86, 7.71, 15.43, 22.71] * 1e-3 J  Tj_loss=[298.15, 398.15] K  Iout_data_loss=[0, 10, 50, 100, 200, 400, 600] A  Eon_scalar=22.86e-3 J  Eoff_scalar=17.14e-3 J  Voff=300 V  Iout_scalar=600 A  diodeModelType=ee.enum.converters.diodeModelType.pwl  diodeTableType=ee.enum.diode.tableType.IfMat  diode_IfMat=[.07, .12, .19, 1.75, 4.24, 7.32, 11.2; .16, .3, .72, 2.14, 4.02, 6.35, 9.12] A  diode_VfMat=[.9, 1.15, 1.25, 1.5, 1.75, 2.17, 2.6, 2.85; .58, .68, .75, 1.1, 1.38, 1.77, 2.27, 2.7] V  diode_TjVec=[25, 125] degC  diode_VfVec=[.5, .7, .9, 1.3, 1.7, 2.1, 2.5] V  diode_IfVec=[.1, .2, .5, 1, 2, 4, 7, 10] A  diode_Vr=-600 V  diode_Ls=150 nH  diode_Erec=0.03 J  thermal_network_parameterization=ee.enum.thermalNetworkTopology.external  Rth=[.03, .2] K/W  Rth_Cauer=[.03, .1, .2] K/W  Rth_Foster=[.03, .2] K/W  thermal_mass_parameterization=ee.enum.thermalNetwork.timeconstant  thermal_mass=[3, 25] J/K  thermal_mass_Cauer=[3, 10, 25] J/K  thermal_mass_Foster=[33, 50] J/K  thermal_time_constant=[.1, 5] s  thermal_time_constant_Cauer=[.1, 1, 5] s  thermal_time_constant_Foster=[1, 10] s  thermal_mass_initial_temperatures=[25, 25] degC  thermal_mass_initial_temperatures_Cauer=[25, 25, 25] degC  junction_thermal_mass=0.1 J/K  steadyState_Foster=simscape.enum.onoff.on  Tvec_initial_Foster=[25, 25, 25, 25] degC  no_thermal_network=0  junction_temperature_specify=off  junction_temperature_priority=None  junction_temperature=25 degC  junction_temperature_nominal_specify=off  junction_temperature_nominal_unit=degC  junction_temperature_nominal_value=1  vT_specify=off  vT_priority=None  vT=0 V  vT_nominal_specify=off  vT_nominal_unit=V  vT_nominal_value=1  Qj_specify=off  Qj_priority=None  Qj=0 W  Qj_nominal_specify=off  Qj_nominal_unit=W  Qj_nominal_value=1
  Current Sensor (Three-Phase) : ee_lib/Sensors & Transducers/Current Sensor (Three-Phase)
      settings: InternalSimscapePortConfiguration="{\"Bottom\":[],\"Left\":[{\"id\":\"a1\",\"label\":\"a1\",\"type\":\"foundation.electrical.electrical\"},{\"id\":\"b1\",\"label\":\"b1\",\"type\":\"foundation.electrical.electrical\"},{\"id\":\"c1\",\"label\":\"c1\",\"type\":\"foundation.electrical.electrical\"}],\"Right\":[{\"id\":\"I_output\",\"label\":\"I\",\"type\":\"output\"},{\"id\":\"a2\",\"label\":\"a2\",\"type\":\"foundation.electrical.electrical\"},{\"id\":\"b2\",\"label\":\"b2\",\"type\":\"foundation.electrical.electrical\"},{\"id\":\"c2\",\"label\":\"c2\",\"type\":\"foundation.electrical.electrical\"}],\"Top\":[]}"
  Gain{4..9} (6 alike) : Gain  Gain=10.0  OutDataTypeStr=double
  Logical Operator : Logic  Operator=NOT  AllPortsSameDT=off  OutDataTypeStr=boolean
  Logical Operator1 : Logic  Operator=NOT  AllPortsSameDT=off  OutDataTypeStr=boolean
  Logical Operator2 : Logic  Operator=NOT  AllPortsSameDT=off  OutDataTypeStr=boolean
  PS-Simulink Converter : nesl_utility/PS-Simulink Converter  PhysicalDomain=network_engine_domain  SubClassName=ps_output  LeftPortType=input  RightPortType=output  PseudoPeriodic=off  Frequencies=[]  VectorFormat=1-D array  Unit=1  AffineConversion=off
  PS-Simulink Converter1 : nesl_utility/PS-Simulink Converter  PhysicalDomain=network_engine_domain  SubClassName=ps_output  LeftPortType=input  RightPortType=output  PseudoPeriodic=off  Frequencies=[]  VectorFormat=1-D array  Unit=1  AffineConversion=off
  Phase Voltage Sensor (Three-Phase) : ee_lib/Sensors & Transducers/Phase Voltage Sensor (Three-Phase)
      settings: SourceProductBaseCode=PS  InternalSimscapePortConfiguration="{\"Bottom\":[],\"Left\":[{\"id\":\"a1\",\"label\":\"a1\",\"type\":\"foundation.electrical.electrical\"},{\"id\":\"b1\",\"label\":\"b1\",\"type\":\"foundation.electrical.electrical\"},{\"id\":\"c1\",\"label\":\"c1\",\"type\":\"foundation.electrical.electrical\"}],\"Right\":[{\"id\":\"V_output\",\"label\":\"V\",\"type\":\"output\"},{\"id\":\"a2\",\"label\":\"a2\",\"type\":\"foundation.electrical.electrical\"},{\"id\":\"b2\",\"label\":\"b2\",\"type\":\"foundation.electrical.electrical\"},{\"id\":\"c2\",\"label\":\"c2\",\"type\":\"foundation.electrical.electrical\"}],\"Top\":[]}"
  Scope1 : Scope  NumInputPorts=3
  Scope16 : Scope  NumInputPorts=6
  Simulink-PS Converter{6..11} (6 alike) : nesl_utility/Simulink-PS Converter  PhysicalDomain=network_engine_domain  SubClassName=ps_input  LeftPortType=input  RightPortType=output  PseudoPeriodic=off  Frequencies=[]  NoiseDistribution=none  NoiseParameters=[]  Unit=1  AffineConversion=off  FilteringAndDerivatives=provide  SimscapeFilterOrder=1  InputFilterTimeConstant=0.001  UdotUserProvided=0
  Solver Configuration : nesl_utility/Solver Configuration  PhysicalDomain=network_engine_domain  SubClassName=solver  LeftPortType=input  RightPortType=generic  Tones=[]  Harmonics=[]  SimulateNoise=off  Profile=off  UseLocalSampling=off  EnableSwitchedLinearOptims=on  FrequencyDomain=off  UseCCode=off  RelTol=0.001  AbsTol=1e-06  MinStep=1e-09  ToWorkspace=off  RevertToSquareIcSolve=off  NumHomotopyIterations=100  PhasorMode=off  PhasorModeNumHarmonics=1  IndexReductionMethod=DerivativeReplacement  DoDC=off  ResidualTolerance=1e-9  UseLocalSolver=on  LocalSolverChoice=NE_BACKWARD_EULER_ADVANCER  LocalSolverSampleTime=Ts  DoFixedCost=on  MaxNonlinIter=4  MaxModeIter=2  ComputeImpulses=off  ImpulseIterations=2  LinearAlgebra=auto  LinearAlgebraNumThread=0  EquationFormulation=NE_TIME_EF  DelaysMemoryBudget=1024  AutomaticFiltering=on  FilteringTimeConstant=0.001  PartitionStorageMethod=AS_NEEDED  PartitionMemoryBudget=1024  PartitionMethod=FAST
      settings: SourceProductBaseCode=SS,PW,VE
  Three-phase currents : Scope
  Three-phase voltages : Scope
  VCC : PMIOPort  Side=Left
  Phase A : PMIOPort  Port=2  Side=Right
  Phase B : PMIOPort  Port=3  Side=Right
  Phase C : PMIOPort  Port=4  Side=Right
  GND : PMIOPort  Port=5  Side=Right
  wires:
  Logical Operator1/1 -> Scope16/2, Gain7/1
  Gain8/1 -> Scope16/1, [AH]
  pwm1/1 -> Gain8/1, Logical Operator1/1, Scope1/1
  pwm2/1 -> Gain6/1, Logical Operator/1, Scope1/2
  pwm3/1 -> Scope1/3, Gain4/1, Logical Operator2/1
  Logical Operator2/1 -> Scope16/6, Gain9/1
  Logical Operator/1 -> Scope16/4, Gain5/1
  Gain6/1 -> Scope16/3, [BH]
  Gain9/1 -> [CL]
  Gain4/1 -> [CH], Scope16/5
  Gain5/1 -> [BL]
  [BL] -> Simulink-PS Converter9/1
  [CH] -> Simulink-PS Converter10/1
  [AL] -> Simulink-PS Converter7/1
  [BH] -> Simulink-PS Converter8/1
  PS-Simulink Converter/1 -> Three-phase currents/1
  [AH] -> Simulink-PS Converter6/1
  Gain7/1 -> [AL]
  [CL] -> Simulink-PS Converter11/1
  PS-Simulink Converter1/1 -> Three-phase voltages/1
  connections:
  Phase Voltage Sensor (Three-Phase)/RConn2 -- Phase Voltage Sensor (Three-Phase)/RConn4 -- Current Sensor (Three-Phase)/LConn3 -- CH (S5)/RConn2 -- CL (S6)/RConn1 -- Phase Voltage Sensor (Three-Phase)/LConn3 -- Phase Voltage Sensor (Three-Phase)/RConn3
  BL (S4)/RConn2 -- CL (S6)/RConn2 -- GND/RConn1 -- AL (S2)/RConn2
  AL (S2)/RConn1 -- AH (S1)/RConn2 -- Current Sensor (Three-Phase)/LConn1 -- Phase Voltage Sensor (Three-Phase)/LConn1
  BL (S4)/RConn1 -- BH (S3)/RConn2 -- Current Sensor (Three-Phase)/LConn2 -- Phase Voltage Sensor (Three-Phase)/LConn2
  AH (S1)/RConn1 -- VCC/RConn1 -- BH (S3)/RConn1 -- CH (S5)/RConn1
  Simulink-PS Converter8/RConn1 -- BH (S3)/LConn1
  Current Sensor (Three-Phase)/RConn1 -- PS-Simulink Converter/LConn1
  Simulink-PS Converter11/RConn1 -- CL (S6)/LConn1
  Simulink-PS Converter6/RConn1 -- AH (S1)/LConn1
  PS-Simulink Converter1/LConn1 -- Phase Voltage Sensor (Three-Phase)/RConn1
  Simulink-PS Converter9/RConn1 -- BL (S4)/LConn1
  Current Sensor (Three-Phase)/RConn2 -- Phase A/RConn1
  Current Sensor (Three-Phase)/RConn3 -- Phase B/RConn1
  Simulink-PS Converter7/RConn1 -- AL (S2)/LConn1
  Current Sensor (Three-Phase)/RConn4 -- Phase C/RConn1
  Simulink-PS Converter10/RConn1 -- CH (S5)/LConn1

== system MotorControl_Bldc/Subsystem1 ==
  Current Sensor : fl_lib/Electrical/Electrical Sensors/Current Sensor
      settings: SourceProductBaseCode=PW,SS,VE
  Current Sensor1 : fl_lib/Electrical/Electrical Sensors/Current Sensor
      settings: SourceProductBaseCode=PW,SS,VE
  Current Sensor2 : fl_lib/Electrical/Electrical Sensors/Current Sensor
      settings: SourceProductBaseCode=PW,SS,VE
  Mux4 : Mux  Inputs=3
  PS-Simulink Converter1 : nesl_utility/PS-Simulink Converter  PhysicalDomain=network_engine_domain  SubClassName=ps_output  LeftPortType=input  RightPortType=output  PseudoPeriodic=off  Frequencies=[]  VectorFormat=1-D array  Unit=A  AffineConversion=off
      settings: SourceProductBaseCode=SS,PW,VE
  PS-Simulink Converter4 : nesl_utility/PS-Simulink Converter  PhysicalDomain=network_engine_domain  SubClassName=ps_output  LeftPortType=input  RightPortType=output  PseudoPeriodic=off  Frequencies=[]  VectorFormat=1-D array  Unit=A  AffineConversion=off
      settings: SourceProductBaseCode=SS,PW,VE
  PS-Simulink Converter5 : nesl_utility/PS-Simulink Converter  PhysicalDomain=network_engine_domain  SubClassName=ps_output  LeftPortType=input  RightPortType=output  PseudoPeriodic=off  Frequencies=[]  VectorFormat=1-D array  Unit=A  AffineConversion=off
      settings: SourceProductBaseCode=SS,PW,VE
  AI : PMIOPort  Side=Left
  BI : PMIOPort  Port=2  Side=Left
  CI : PMIOPort  Port=3  Side=Left
  AO : PMIOPort  Port=4  Side=Right
  CO : PMIOPort  Port=5  Side=Right
  BO : PMIOPort  Port=6  Side=Right
  Out1 : Outport
  wires:
  PS-Simulink Converter5/1 -> Mux4/2
  PS-Simulink Converter4/1 -> Mux4/1
  Mux4/1 -> Out1/1
  PS-Simulink Converter1/1 -> Mux4/3
  connections:
  PS-Simulink Converter4/LConn1 -- Current Sensor/RConn1
  Current Sensor1/RConn2 -- BO/RConn1
  Current Sensor2/LConn1 -- CI/RConn1
  PS-Simulink Converter5/LConn1 -- Current Sensor1/RConn1
  PS-Simulink Converter1/LConn1 -- Current Sensor2/RConn1
  Current Sensor1/LConn1 -- BI/RConn1
  Current Sensor/RConn2 -- AO/RConn1
  Current Sensor/LConn1 -- AI/RConn1
  Current Sensor2/RConn2 -- CO/RConn1

== system MotorControl_Bldc/Subsystem10 ==
  Mux4 : Mux  Inputs=3
  PS-Simulink Converter : nesl_utility/PS-Simulink Converter  PhysicalDomain=network_engine_domain  SubClassName=ps_output  LeftPortType=input  RightPortType=output  PseudoPeriodic=off  Frequencies=[]  VectorFormat=inherit  Unit=inherit  AffineConversion=off
      settings: SourceProductBaseCode=SS,PW,VE
  PS-Simulink Converter1 : nesl_utility/PS-Simulink Converter  PhysicalDomain=network_engine_domain  SubClassName=ps_output  LeftPortType=input  RightPortType=output  PseudoPeriodic=off  Frequencies=[]  VectorFormat=1-D array  Unit=V  AffineConversion=off
      settings: SourceProductBaseCode=SS,PW,VE
  PS-Simulink Converter2 : nesl_utility/PS-Simulink Converter  PhysicalDomain=network_engine_domain  SubClassName=ps_output  LeftPortType=input  RightPortType=output  PseudoPeriodic=off  Frequencies=[]  VectorFormat=1-D array  Unit=V  AffineConversion=off
      settings: SourceProductBaseCode=SS,PW,VE
  Voltage Sensor1 : fl_lib/Electrical/Electrical Sensors/Voltage Sensor
      settings: SourceProductBaseCode=PW,SS,VE
  Voltage Sensor2 : fl_lib/Electrical/Electrical Sensors/Voltage Sensor
      settings: SourceProductBaseCode=PW,SS,VE
  Voltage Sensor3 : fl_lib/Electrical/Electrical Sensors/Voltage Sensor
      settings: SourceProductBaseCode=PW,SS,VE
  AV : PMIOPort  Side=Left
  BV : PMIOPort  Port=2  Side=Left
  CV : PMIOPort  Port=3  Side=Left
  GND : PMIOPort  Port=4  Side=Left
  OUT : Outport
  wires:
  PS-Simulink Converter/1 -> Mux4/3
  PS-Simulink Converter1/1 -> Mux4/1
  PS-Simulink Converter2/1 -> Mux4/2
  Mux4/1 -> OUT/1
  connections:
  Voltage Sensor2/RConn2 -- GND/RConn1 -- Voltage Sensor3/RConn2 -- Voltage Sensor1/RConn2
  PS-Simulink Converter1/LConn1 -- Voltage Sensor1/RConn1
  Voltage Sensor3/LConn1 -- CV/RConn1
  PS-Simulink Converter2/LConn1 -- Voltage Sensor2/RConn1
  Voltage Sensor1/LConn1 -- AV/RConn1
  PS-Simulink Converter/LConn1 -- Voltage Sensor3/RConn1
  Voltage Sensor2/LConn1 -- BV/RConn1

== system MotorControl_Bldc/Subsystem11 ==
  Mux4 : Mux  Inputs=3
  PS-Simulink Converter : nesl_utility/PS-Simulink Converter  PhysicalDomain=network_engine_domain  SubClassName=ps_output  LeftPortType=input  RightPortType=output  PseudoPeriodic=off  Frequencies=[]  VectorFormat=inherit  Unit=inherit  AffineConversion=off
      settings: SourceProductBaseCode=SS,PW,VE
  PS-Simulink Converter1 : nesl_utility/PS-Simulink Converter  PhysicalDomain=network_engine_domain  SubClassName=ps_output  LeftPortType=input  RightPortType=output  PseudoPeriodic=off  Frequencies=[]  VectorFormat=1-D array  Unit=V  AffineConversion=off
      settings: SourceProductBaseCode=SS,PW,VE
  PS-Simulink Converter2 : nesl_utility/PS-Simulink Converter  PhysicalDomain=network_engine_domain  SubClassName=ps_output  LeftPortType=input  RightPortType=output  PseudoPeriodic=off  Frequencies=[]  VectorFormat=1-D array  Unit=V  AffineConversion=off
      settings: SourceProductBaseCode=SS,PW,VE
  Voltage Sensor1 : fl_lib/Electrical/Electrical Sensors/Voltage Sensor
      settings: SourceProductBaseCode=PW,SS,VE
  Voltage Sensor2 : fl_lib/Electrical/Electrical Sensors/Voltage Sensor
      settings: SourceProductBaseCode=PW,SS,VE
  Voltage Sensor3 : fl_lib/Electrical/Electrical Sensors/Voltage Sensor
      settings: SourceProductBaseCode=PW,SS,VE
  AV : PMIOPort  Side=Left
  BV : PMIOPort  Port=2  Side=Left
  CV : PMIOPort  Port=3  Side=Left
  GND : PMIOPort  Port=4  Side=Left
  OUT : Outport
  wires:
  PS-Simulink Converter/1 -> Mux4/3
  PS-Simulink Converter1/1 -> Mux4/1
  PS-Simulink Converter2/1 -> Mux4/2
  Mux4/1 -> OUT/1
  connections:
  Voltage Sensor3/RConn2 -- Voltage Sensor1/RConn2 -- Voltage Sensor2/RConn2 -- GND/RConn1
  PS-Simulink Converter1/LConn1 -- Voltage Sensor1/RConn1
  Voltage Sensor3/LConn1 -- CV/RConn1
  PS-Simulink Converter2/LConn1 -- Voltage Sensor2/RConn1
  Voltage Sensor1/LConn1 -- AV/RConn1
  PS-Simulink Converter/LConn1 -- Voltage Sensor3/RConn1
  Voltage Sensor2/LConn1 -- BV/RConn1
